simulink model "MultiSizeCells"  (R2020b)
settings: Solver=ode45  StartTime=0.0  StopTime=2  RelTol=1e-3  EnableMultiTasking=on
libraries: NeuroModelerLibrary x6
settings Model: Creator=Bakhshiev  LastModifiedBy=Bakhshiev
settings DataIOCC: LimitDataPoints=on  SaveFormat=Array  SignalLoggingSaveFormat=ModelDataLogs  ReturnWorkspaceOutputs=off
settings OptimizationCC: ExpressionDepthLimit=2147483647  InitFltsAndDblsToZero=on  LifeSpan=inf
settings DebuggingCC: UnderspecifiedInitializationDetection=Classic  MergeDetectMultiDrivingBlocksExec=none  SolverPrmCheckMsg=warning  FcnCallInpInsideContextMsg=warning  StateNameClashWarn=warning  SFUnexpectedBacktrackingDiag=warning  SFNoUnconditionalDefaultTransitionDiag=warning  SFExecutionAtInitializationDiag=none  ArithmeticOperatorsInVariantConditions=warning
settings HardwareCC: ProdBitPerPointer=32  ProdBitPerSizeT=32  ProdBitPerPtrDiffT=32  ProdLargestAtomicFloat=None  ProdIntDivRoundTo=Undefined  ProdEndianess=Unspecified  ProdWordSize=32  ProdHWDeviceType=32-bit Generic
settings ModelReferenceCC: PropagateSignalLabelsOutOfModel=off
settings SFSimCC: CustomCodeUndefinedFunction=UseInterfaceOnly
settings CodeAppCC: StateflowObjectComments=on
settings GRTTargetCC: TargetLangStandard=C89/C90 (ANSI)  CombineOutputUpdateFcns=off  GRTInterface=on
settings ConfigComp: CovMetricSettings=dw  CovSaveCumulativeToWorkspaceVar=on  CovSaveSingleToWorkspaceVar=on

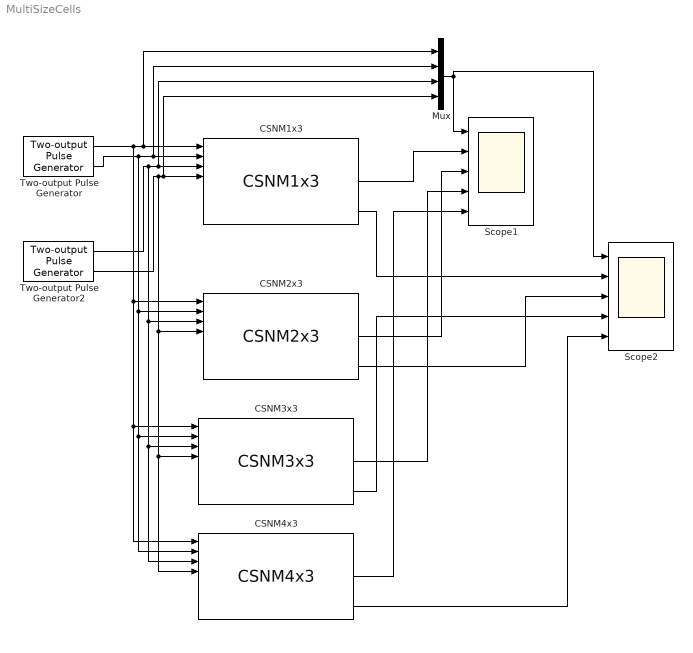
== system MultiSizeCells ==
  CSNM1x3 : NeuroModelerLibrary/CSNM/CSNM1x3  SystemSampleTime=-1  VariantActivationTime=update diagram  Latency=0  AutoFrameSizeCalculation=off
      link override LTZoneV2: T=1
  CSNM2x3 : NeuroModelerLibrary/CSNM/CSNM2x3  SystemSampleTime=-1  VariantActivationTime=update diagram  Latency=0  AutoFrameSizeCalculation=off
      link override LTZoneV2: T=1
  CSNM3x3 : NeuroModelerLibrary/CSNM/CSNM3x3  SystemSampleTime=-1  VariantActivationTime=update diagram  Latency=0  AutoFrameSizeCalculation=off
      link override LTZoneV2: T=1
  CSNM4x3 : NeuroModelerLibrary/CSNM/CSNM4x3  SystemSampleTime=-1  VariantActivationTime=update diagram  Latency=0  AutoFrameSizeCalculation=off
      link override LTZoneV2: T=1
  Mux : Mux
  Scope1 : Scope  NumInputPorts=5
  Scope2 : Scope  NumInputPorts=5
  Two-output Pulse Generator : NeuroModelerLibrary/Support/Two-output Pulse Generator  A=1  P1=200  P2=200  PW=1  ST=0.001  OOn1=0.5  OOff1=0.6  OOn2=0.8  OOff2=0.9
  Two-output Pulse Generator2 : NeuroModelerLibrary/Support/Two-output Pulse Generator  A=1  P1=200  P2=200  PW=1  ST=0.001  OOn1=1.2  OOff1=1.3  OOn2=1.6  OOff2=1.7
  wires:
  Two-output Pulse Generator/1 -> CSNM1x3/1, Mux/1, CSNM4x3/1, CSNM3x3/1, CSNM2x3/1
  Two-output Pulse Generator/2 -> CSNM1x3/2, Mux/2, CSNM4x3/2, CSNM3x3/2, CSNM2x3/2
  Mux/1 -> Scope2/1, Scope1/1
  Two-output Pulse Generator2/2 -> CSNM1x3/4, Mux/4, CSNM4x3/4, CSNM3x3/4, CSNM2x3/4
  Two-output Pulse Generator2/1 -> CSNM1x3/3, Mux/3, CSNM4x3/3, CSNM3x3/3, CSNM2x3/3
  CSNM1x3/2 -> Scope1/2
  CSNM2x3/2 -> Scope1/3
  CSNM3x3/2 -> Scope1/4
  CSNM4x3/2 -> Scope1/5
  CSNM1x3/3 -> Scope2/2
  CSNM2x3/3 -> Scope2/3
  CSNM3x3/3 -> Scope2/4
  CSNM4x3/3 -> Scope2/5
